simulink model "ControlEngineeringSimulink"  (R2020a)
settings: Solver=FixedStepAuto  StartTime=0.0  StopTime=50  FixedStep=1/8000  RelTol=1e-3
values from neighbouring files (symbols this model uses):
  A = [0 1 0 0 ... (first row only)    [ControllerToProject.m]
  B = [0 0 ... (first row only)    [ControllerToProject.m]
  C = [1 0 0 0 ... (first row only)    [ControllerToProject.m]
  g = 9.81    [ControllerToProject.m]    (also in Parameters.m = 9.82)
  l = 0.36022    [ControllerToProject.m]    (also in Parameters.m = 0.35)
  mc = 0.9+0.1    (= 1)    [ControllerToProject.m]    (also in Parameters.m = 0.9)
  mp = 0.08887    [ControllerToProject.m]    (also in Parameters.m = 0.1)
undefined symbols (not defined in the file or in its folder): bc, F, Fi, L, M, sigbuilder_block
libraries: simulink x4
settings Model: Creator=Emil  LastModifiedBy=Emil
settings SolverCC: ZeroCrossAlgorithm=Adaptive  AlgebraicLoopSolver=LineSearch
settings DebuggingCC: IgnoredZcDiagnostic=none

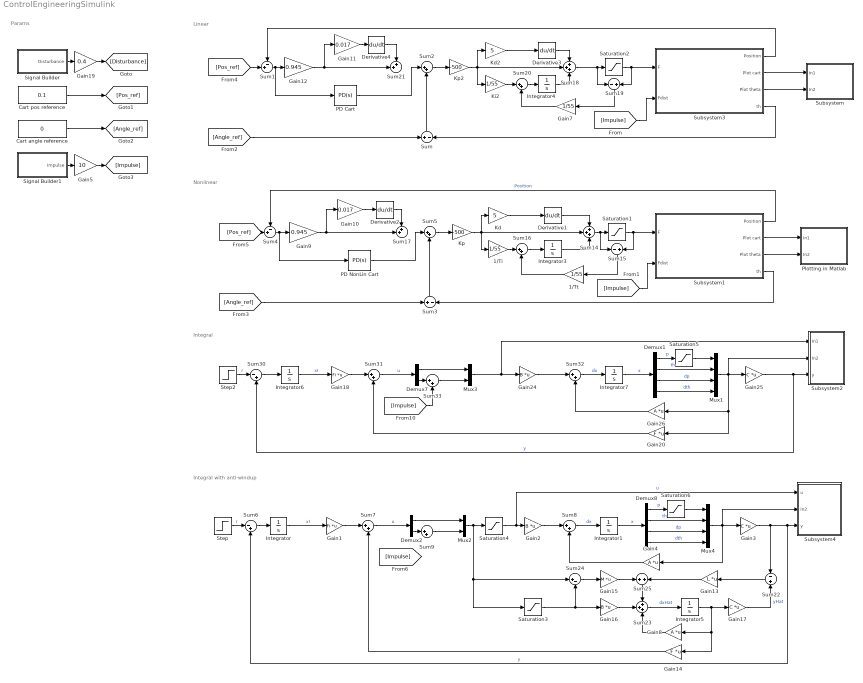
== system ControlEngineeringSimulink ==
  note: Params
  note: Nonlinear
  note: Linear
  note: Integral with anti-windup
  note: Integral
  1/Ti : Gain  Gain=1/55
  1/Tt : Gain  Gain=1/55
  Cart angle reference : Constant  Value=0
  Cart pos reference : Constant  Value=0.1
  Demux1 : Demux
  Demux2 : Demux  Outputs=2
  Demux7 : Demux  Outputs=2
  Demux8 : Demux
  Derivative{1..4} (4 alike) : Derivative
  Gain1 : Gain  Gain=Fi  Multiplication=Matrix(K*u)
  Gain10 : Gain  Gain=0.017
  Gain11 : Gain  Gain=0.017
  Gain12 : Gain  Gain=0.945
  Gain13 : Gain  Gain=L  Multiplication=Matrix(K*u)
  Gain14 : Gain  Gain=F  Multiplication=Matrix(K*u)
  Gain15 : Gain  Gain=M  Multiplication=Matrix(K*u)
  Gain16 : Gain  Gain=B  Multiplication=Matrix(K*u)
  Gain17 : Gain  Gain=C  Multiplication=Matrix(K*u)
  Gain18 : Gain  Gain=Fi  Multiplication=Matrix(K*u)
  Gain19 : Gain  Gain=0.4
  Gain2 : Gain  Gain=B  Multiplication=Matrix(K*u)
  Gain20 : Gain  Gain=F  Multiplication=Matrix(K*u)
  Gain24 : Gain  Gain=B  Multiplication=Matrix(K*u)
  Gain25 : Gain  Gain=C  Multiplication=Matrix(K*u)
  Gain26 : Gain  Gain=A  Multiplication=Matrix(K*u)
  Gain3 : Gain  Gain=C  Multiplication=Matrix(K*u)
  Gain4 : Gain  Gain=A  Multiplication=Matrix(K*u)
  Gain5 : Gain  Gain=10
  Gain7 : Gain  Gain=1/55
  Gain8 : Gain  Gain=A  Multiplication=Matrix(K*u)
  Gain9 : Gain  Gain=0.945
  Integrator{,1,3..7} (7 alike) : Integrator
  Kd : Gain  Gain=5
  Kd2 : Gain  Gain=5
  Ki2 : Gain  Gain=1/55
  Kp : Gain  Gain=-500
  Kp2 : Gain  Gain=-500
  Mux1 : Mux
  Mux2 : Mux  Inputs=2
  Mux3 : Mux  Inputs=2
  Mux4 : Mux
  PD Cart : simulink/Continuous/PID Controller  Controller=PD  Form=Ideal  TimeDomain=Continuous-time  UseExternalTs=off  SampleTime=-1  IntegratorMethod=Forward Euler  FilterMethod=Forward Euler  ControllerParametersSource=internal  P=0.945  I=0  D=0.017  UseFilter=on  N=20  TunerSelectOption=Transfer Function Based (PID Tuner App)  InitialConditionSource=internal  InitialConditionForIntegrator=0  InitialConditionForFilter=0  DifferentiatorICPrevScaledInput=0  ExternalReset=none  TrackingMode=off  Kt=1  LimitOutput=off  UpperSaturationLimit=inf  LowerSaturationLimit=-inf  LinearizeAsGain=on  AntiWindupMode=none  Kb=1  POutMin=[]  POutMax=[]  IOutMin=[]  IOutMax=[]  DOutMin=[]  DOutMax=[]  NOutMin=[]  NOutMax=[]  SumOutMin=[]  SumOutMax=[]  SaturationOutMin=[]  SaturationOutMax=[]  PParamMin=[]  PParamMax=[]  IParamMin=[]  IParamMax=[]  DParamMin=[]  DParamMax=[]  NParamMin=[]  NParamMax=[]  KbParamMin=[]  KbParamMax=[]  KtParamMin=[]  KtParamMax=[]  KbOutMin=[]  KbOutMax=[]  KtOutMin=[]  KtOutMax=[]  IntegratorOutMin=[]  IntegratorOutMax=[]  FilterOutMin=[]  FilterOutMax=[]  SumI1OutMin=[]  SumI1OutMax=[]  SumI2OutMin=[]  SumI2OutMax=[]  SumI3OutMin=[]  SumI3OutMax=[]  SumI4OutMin=[]  SumI4OutMax=[]  SumDOutMin=[]  SumDOutMax=[]  DifferentiatorOutMin=[]  DifferentiatorOutMax=[]  FilterDiffOutCoefMin=[]  FilterDiffOutCoefMax=[]  ReciprocalOutMin=[]  ReciprocalOutMax=[]  SumDenOutMin=[]  SumDenOutMax=[]  SumNumOutMin=[]  SumNumOutMax=[]  DivideOutMin=[]  DivideOutMax=[]  UdiffTsProdOutMin=[]  UdiffTsProdOutMax=[]  NTsProdOutMin=[]  NTsProdOutMax=[]  UintegralTsProdOutMin=[]  UintegralTsProdOutMax=[]  UngainTsProdOutMin=[]  UngainTsProdOutMax=[]  IntegratorContinuousStateAttributes=''  IntegratorStateMustResolveToSignalObject=off  IntegratorRTWStateStorageClass=Auto  FilterContinuousStateAttributes=''  FilterStateMustResolveToSignalObject=off  FilterRTWStateStorageClass=Auto  ParallelPVariant=Passthrough  IdealPVariant=InternalParameters  IVariant=Disabled  DVariant=InternalParameters  IntegratorVariant=Disabled  SatVariant=Disabled  AWVariant=Disabled  PCopyVariant=Disabled  TRVariant=Disabled  FdbkBlocksVariant=Forward  IdealPFdbkVariant=Disabled  SatFdbkVariant=Disabled  DerivativeFilterVariant=ContFilter  NVariant=InternalParameters  NCopyVariant=Disabled  FilterICVariant=InternalICsFilter  IntegratorICVariant=Disabled  ExternalResetVariant=Disabled  TRSumVariant=Passthrough  SumFdbkVariant=Disabled  SumVariant=Sum_PD  TsampFilterVariant=InternalTs  TsampNgainVariant=Passthrough  TsampIntegralVariant=Disabled_SignalSpec
  PD NonLin Cart : simulink/Continuous/PID Controller  Controller=PD  Form=Ideal  TimeDomain=Continuous-time  UseExternalTs=off  SampleTime=-1  IntegratorMethod=Forward Euler  FilterMethod=Forward Euler  ControllerParametersSource=internal  P=0.945  I=0  D=0.017  UseFilter=on  N=20  TunerSelectOption=Transfer Function Based (PID Tuner App)  InitialConditionSource=internal  InitialConditionForIntegrator=0  InitialConditionForFilter=0  DifferentiatorICPrevScaledInput=0  ExternalReset=none  TrackingMode=off  Kt=1  LimitOutput=off  UpperSaturationLimit=inf  LowerSaturationLimit=-inf  LinearizeAsGain=on  AntiWindupMode=none  Kb=1  POutMin=[]  POutMax=[]  IOutMin=[]  IOutMax=[]  DOutMin=[]  DOutMax=[]  NOutMin=[]  NOutMax=[]  SumOutMin=[]  SumOutMax=[]  SaturationOutMin=[]  SaturationOutMax=[]  PParamMin=[]  PParamMax=[]  IParamMin=[]  IParamMax=[]  DParamMin=[]  DParamMax=[]  NParamMin=[]  NParamMax=[]  KbParamMin=[]  KbParamMax=[]  KtParamMin=[]  KtParamMax=[]  KbOutMin=[]  KbOutMax=[]  KtOutMin=[]  KtOutMax=[]  IntegratorOutMin=[]  IntegratorOutMax=[]  FilterOutMin=[]  FilterOutMax=[]  SumI1OutMin=[]  SumI1OutMax=[]  SumI2OutMin=[]  SumI2OutMax=[]  SumI3OutMin=[]  SumI3OutMax=[]  SumI4OutMin=[]  SumI4OutMax=[]  SumDOutMin=[]  SumDOutMax=[]  DifferentiatorOutMin=[]  DifferentiatorOutMax=[]  FilterDiffOutCoefMin=[]  FilterDiffOutCoefMax=[]  ReciprocalOutMin=[]  ReciprocalOutMax=[]  SumDenOutMin=[]  SumDenOutMax=[]  SumNumOutMin=[]  SumNumOutMax=[]  DivideOutMin=[]  DivideOutMax=[]  UdiffTsProdOutMin=[]  UdiffTsProdOutMax=[]  NTsProdOutMin=[]  NTsProdOutMax=[]  UintegralTsProdOutMin=[]  UintegralTsProdOutMax=[]  UngainTsProdOutMin=[]  UngainTsProdOutMax=[]  IntegratorContinuousStateAttributes=''  IntegratorStateMustResolveToSignalObject=off  IntegratorRTWStateStorageClass=Auto  FilterContinuousStateAttributes=''  FilterStateMustResolveToSignalObject=off  FilterRTWStateStorageClass=Auto  ParallelPVariant=Passthrough  IdealPVariant=InternalParameters  IVariant=Disabled  DVariant=InternalParameters  IntegratorVariant=Disabled  SatVariant=Disabled  AWVariant=Disabled  PCopyVariant=Disabled  TRVariant=Disabled  FdbkBlocksVariant=Forward  IdealPFdbkVariant=Disabled  SatFdbkVariant=Disabled  DerivativeFilterVariant=ContFilter  NVariant=InternalParameters  NCopyVariant=Disabled  FilterICVariant=InternalICsFilter  IntegratorICVariant=Disabled  ExternalResetVariant=Disabled  TRSumVariant=Passthrough  SumFdbkVariant=Disabled  SumVariant=Sum_PD  TsampFilterVariant=InternalTs  TsampNgainVariant=Passthrough  TsampIntegralVariant=Disabled_SignalSpec
  Plotting in Matlab : Subsystem
  Saturation{1..4} (4 alike) : Saturate  UpperLimit=50  LowerLimit=-50
  Saturation5 : Saturate  UpperLimit=0.8  LowerLimit=-0.8
  Saturation6 : Saturate  UpperLimit=0.8  LowerLimit=-0.8
  Signal Builder : Subsystem  Tag=STV Subsys  LoadFcn=sigbuilder_block('load');  StartFcn=sigbuilder_block('start');  StopFcn=sigbuilder_block('stop');  ClipboardFcn=sigbuilder_block('clipboard');  mask(Sigbuilder block){tuvar=[0:10]}
      mask help: Simulink:masks:SigbuilderBlock_MD
      mask init:
      | if ~strcmp(get_param(bdroot(gcbh),'SimulationStatus'),'stopped') tuvar = sigbuilder_block('maskInit'); end
      settings: CopyFcn=sigbuilder_block('copy');  DeleteFcn=sigbuilder_block('delete');  ModelCloseFcn=sigbuilder_block('modelClose');  PreSaveFcn=sigbuilder_block('preSave');  PauseFcn=sigbuilder_block('pause');  ContinueFcn=sigbuilder_block('continue');  NameChangeFcn=sigbuilder_block('namechange');  OpenFcn=sigbuilder_block('open',[3.75 670.5 818.25 342 ]);  CloseFcn=sigbuilder_block('close');
      mask Display: plot(0, 0, 100, 100,[2, 2, 32, 32, 2], [68, 8, 8, 68, 68],[32, 2], [38, 38], [32, 19, 2],[53, 60, 44], [32, 17, 17, 2],[16, 16, 31, 31]);txt = getActiveGroup(gcbh);text(2, 100, txt,'verticalAlignment', 'top');
  Signal Builder1 : Subsystem  Tag=STV Subsys  LoadFcn=sigbuilder_block('load');  StartFcn=sigbuilder_block('start');  StopFcn=sigbuilder_block('stop');  ClipboardFcn=sigbuilder_block('clipboard');  mask(Sigbuilder block){tuvar=[0:10]}
      mask help: Simulink:masks:SigbuilderBlock_MD
      mask init:
      | if ~strcmp(get_param(bdroot(gcbh),'SimulationStatus'),'stopped') tuvar = sigbuilder_block('maskInit'); end
      settings: CopyFcn=sigbuilder_block('copy');  DeleteFcn=sigbuilder_block('delete');  ModelCloseFcn=sigbuilder_block('modelClose');  PreSaveFcn=sigbuilder_block('preSave');  PauseFcn=sigbuilder_block('pause');  ContinueFcn=sigbuilder_block('continue');  NameChangeFcn=sigbuilder_block('namechange');  OpenFcn=sigbuilder_block('open',[437.6 199.2 550.4 400 ]);  CloseFcn=sigbuilder_block('close');
      mask Display: plot(0, 0, 100, 100,[2, 2, 32, 32, 2], [68, 8, 8, 68, 68],[32, 2], [38, 38], [32, 19, 2],[53, 60, 44], [32, 17, 17, 2],[16, 16, 31, 31]);txt = getActiveGroup(gcbh);text(2, 100, txt,'verticalAlignment', 'top');
  Step : Step  Time=0  Before=[0, 0]  After=[0, 0.1]  SampleTime=0
  Step2 : Step  Time=0  Before=[0, 0]  After=[0, 0.1]  SampleTime=0
  Subsystem : Subsystem
  Subsystem1 : Subsystem
      mask Display: image('System.png'); % Use "Edit Image" on toolstrip to change.
  Subsystem2 : Subsystem
  Subsystem3 : Subsystem
      mask Display: image('System.png'); % Use "Edit Image" on toolstrip to change.
  Subsystem4 : Subsystem
  Sum : Sum  Inputs=+-
  Sum1 : Sum  Inputs=-+|
  Sum14 : Sum  Inputs=+++
  Sum15 : Sum  Inputs=-+
  Sum{2,5,7..9,16,20,31..33} (10 alike) : Sum  Inputs=|++
  Sum17 : Sum  Inputs=++|
  Sum18 : Sum  Inputs=+++
  Sum19 : Sum  Inputs=-+
  Sum21 : Sum  Inputs=++|
  Sum22 : Sum  Inputs=-+
  Sum23 : Sum  Inputs=+++
  Sum24 : Sum  Inputs=|+-
  Sum25 : Sum
  Sum3 : Sum  Inputs=+-
  Sum30 : Sum  Inputs=|-+
  Sum4 : Sum  Inputs=-+|
  Sum6 : Sum  Inputs=|-+
  wires:
  Subsystem3/1(Position) -> Sum1/1
  Subsystem3/4(th) -> Sum/2
  [Angle_ref] -> Sum/1
  [Pos_ref] -> Sum1/2
  Sum/1 -> Sum2/2
  [Pos_ref] -> Sum4/2
  [Angle_ref] -> Sum3/1
  Sum3/1 -> Sum5/2
  Subsystem1/1(Position) -> Sum4/1  "Position"
  Subsystem1/4(th) -> Sum3/2
  Cart pos reference/1 -> [Pos_ref]
  Cart angle reference/1 -> [Angle_ref]
  Sum6/1 -> Integrator/1
  Gain3/1 -> Sum22/1, Sum6/2, Subsystem4/3(y)  "y"
  Gain1/1 -> Sum7/1
  Gain2/1 -> Sum8/1
  Step/1 -> Sum6/1  "r"
  Gain4/1 -> Sum8/2
  Mux4/1 -> Gain4/1, Subsystem4/2(In2), Gain3/1
  Integrator/1 -> Gain1/1  "xI"
  Sum9/1 -> Mux2/2
  Sum7/1 -> Demux2/1  "u"
  Mux2/1 -> Saturation3/1, Sum24/1, Saturation4/1
  Demux2/1 -> Mux2/1
  Sum8/1 -> Integrator1/1  "dx"
  Kp/1 -> 1/Ti/1, Sum14/2, Kd/1
  Integrator3/1 -> Sum14/3
  Derivative1/1 -> Sum14/1
  Saturation1/1 -> Subsystem1/1(F), Sum15/2
  Kd/1 -> Derivative1/1
  1/Ti/1 -> Sum16/1
  Sum16/1 -> Integrator3/1
  Derivative2/1 -> Sum17/1
  Sum14/1 -> Sum15/1, Saturation1/1
  Sum15/1 -> 1/Tt/1
  1/Tt/1 -> Sum16/2
  Gain9/1 -> Gain10/1, Sum17/2
  Sum19/1 -> Gain7/1
  Gain7/1 -> Sum20/2
  Sum18/1 -> Sum19/1, Saturation2/1
  Sum2/1 -> Kp2/1
  Kd2/1 -> Derivative3/1
  Ki2/1 -> Sum20/1
  Sum20/1 -> Integrator4/1
  Saturation2/1 -> Sum19/2, Subsystem3/1(F)
  Integrator4/1 -> Sum18/3
  Derivative3/1 -> Sum18/1
  Kp2/1 -> Ki2/1, Sum18/2, Kd2/1
  Gain11/1 -> Derivative4/1
  Gain12/1 -> Sum21/2, Gain11/1
  Derivative4/1 -> Sum21/1
  Gain15/1 -> Sum25/1
  Integrator5/1 -> Gain14/1, Gain8/1, Gain17/1
  Saturation3/1 -> Gain16/1, Sum24/2
  Gain14/1 -> Sum7/2
  Saturation4/1 -> Subsystem4/1(u), Gain2/1  "u"
  Sum24/1 -> Gain15/1
  Gain13/1 -> Sum25/2
  Gain17/1 -> Sum22/2  "yHat"
  Sum25/1 -> Sum23/1
  Sum23/1 -> Integrator5/1  "dxHat"
  Gain8/1 -> Sum23/3
  Gain16/1 -> Sum23/2
  Sum22/1 -> Gain13/1
  Gain10/1 -> Derivative2/1
  Sum5/1 -> Kp/1
  Sum4/1 -> PD NonLin Cart/1, Gain9/1
  Demux1/1 -> Saturation5/1  "p"
  Demux1/3 -> Mux1/3  "dp"
  Integrator7/1 -> Demux1/1  "x"
  Gain25/1 -> Sum30/2, Subsystem2/3(y)  "y"
  Gain26/1 -> Sum32/2
  Demux7/2 -> Sum33/1
  Gain24/1 -> Sum32/1
  Sum33/1 -> Mux3/2
  Sum31/1 -> Demux7/1  "u"
  Sum30/1 -> Integrator6/1
  Demux1/4 -> Mux1/4  "dth"
  Mux3/1 -> Subsystem2/1(In1), Gain24/1
  Mux1/1 -> Gain20/1, Gain26/1, Subsystem2/2(In2), Gain25/1
  Integrator6/1 -> Gain18/1  "xI"
  Sum32/1 -> Integrator7/1  "dx"
  Demux7/1 -> Mux3/1
  Gain18/1 -> Sum31/1
  Step2/1 -> Sum30/1  "r"
  Gain20/1 -> Sum31/2
  Saturation5/1 -> Mux1/1
  Demux1/2 -> Mux1/2  "th"
  Demux8/4 -> Mux4/4  "dth"
  Demux8/3 -> Mux4/3  "dp"
  Demux8/2 -> Mux4/2  "th"
  Integrator1/1 -> Demux8/1  "x"
  Saturation6/1 -> Mux4/1
  Demux8/1 -> Saturation6/1  "p"
  Signal Builder/1(Disturbance) -> Gain19/1
  Gain19/1 -> [Disturbance]
  Demux2/2 -> Sum9/1
  Signal Builder1/1(Impulse) -> Gain5/1
  Gain5/1 -> [Impulse]
  [Impulse] -> Subsystem3/2(Fdist)
  [Impulse] -> Subsystem1/2(Fdist)
  Subsystem1/2(Plot cart) -> Plotting in Matlab/1(In1)
  Subsystem1/3(Plot theta) -> Plotting in Matlab/2(In2)
  Subsystem3/2(Plot cart) -> Subsystem/1(In1)
  Subsystem3/3(Plot theta) -> Subsystem/2(In2)
  Sum1/1 -> PD Cart/1, Gain12/1
  PD Cart/1 -> Sum2/1
  PD NonLin Cart/1 -> Sum5/1
  [Impulse] -> Sum33/2

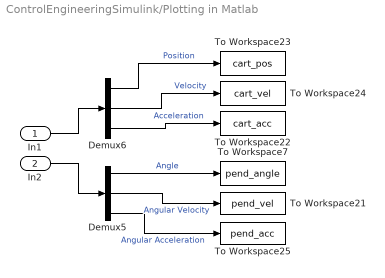
== system ControlEngineeringSimulink/Plotting in Matlab ==
  In1 : Inport
  In2 : Inport  Port=2
  Demux5 : Demux  Outputs=3
  Demux6 : Demux  Outputs=3
  To Workspace21 : ToWorkspace  VariableName=pend_vel  SaveFormat=Timeseries  SampleTime=-1
  To Workspace22 : ToWorkspace  VariableName=cart_acc  SaveFormat=Timeseries  SampleTime=-1
  To Workspace23 : ToWorkspace  VariableName=cart_pos  SaveFormat=Timeseries  SampleTime=-1
  To Workspace24 : ToWorkspace  VariableName=cart_vel  SaveFormat=Timeseries  SampleTime=-1
  To Workspace25 : ToWorkspace  VariableName=pend_acc  SaveFormat=Timeseries  SampleTime=-1
  To Workspace7 : ToWorkspace  VariableName=pend_angle  SaveFormat=Timeseries  SampleTime=-1
  wires:
  In1/1 -> Demux6/1
  Demux5/1 -> To Workspace7/1  "Angle"
  In2/1 -> Demux5/1
  Demux5/2 -> To Workspace21/1  "Angular Velocity"
  Demux6/1 -> To Workspace23/1  "Position"
  Demux5/3 -> To Workspace25/1  "Angular Acceleration"
  Demux6/2 -> To Workspace24/1  "Velocity"
  Demux6/3 -> To Workspace22/1  "Acceleration"

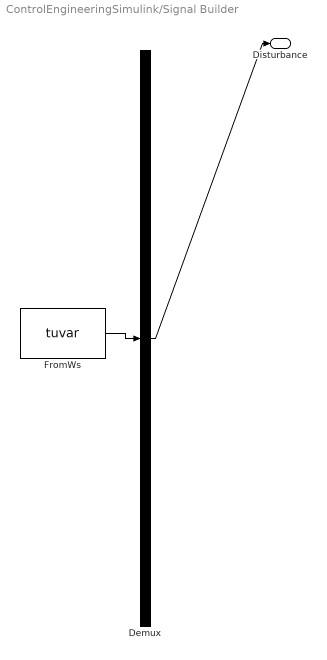
== system ControlEngineeringSimulink/Signal Builder ==
  Demux : Demux  Tag=STV Demux  Outputs=1
      settings: DisplayOption=none
  FromWs : FromWorkspace  Tag=STV FromWs  VariableName=tuvar
      SigBuilderData=|
      | common.afterFinalStr = 'Extrapolate'
      | common.sampleTime = 0
      | dataSet.timeRange = [0 10]
      | dataSet.name = 'Group 1'
      | sbobj.Groups.Name = 'Group 1'
      | sbobj.Groups.Signals.Name = 'Disturbance'
      | sbobj.Groups.Signals.XData = [0 0.25 0.5 0.75 1 1.25 1.5 1.75 2 2.25 2.5 2.75 3 3.25 3.5 3.75 4 4.25 4.5 4.75 5 5.25 5.5 5.75 6 6.25 6.5 6.75 7 7.25 7.5 7.75 8 8.25 8.5 8.75 9 9.25 9.5 9.75 10]
      | sbobj.Groups.Signals.YData = [0 0 0 0 0 0 0 0 0 0 0 -2.77555756156e-17 -0.002 0.063 0.002 -0.03 -0.05 -0.05 0.01 -0.146 0.16 0.08 0.1 0.089 0.193 0.06 0.02 -2.7756e-18 -0.022 -0.034 -0.099 -0.084 -0.01 -0.02 -0.051 -0.045 0.02 0.02 0.176 -2.7756e-18 -2.77555756156e-17]
  Disturbance : Outport  Tag=STV Outport
  wires:
  FromWs/1 -> Demux/1
  Demux/1 -> Disturbance/1

== system ControlEngineeringSimulink/Signal Builder1 ==
  Demux : Demux  Tag=STV Demux  Outputs=1
      settings: DisplayOption=none
  FromWs : FromWorkspace  Tag=STV FromWs  VariableName=tuvar
      SigBuilderData=|
      | common.afterFinalStr = 'Extrapolate'
      | common.sampleTime = 0
      | dataSet.timeRange = [0 10]
      | dataSet.name = 'Group 1'
      | sbobj.Groups.Name = 'Group 1'
      | sbobj.Groups.Signals.Name = 'Impulse'
      | sbobj.Groups.Signals.XData = [0 0.1 0.2 10]
      | sbobj.Groups.Signals.YData = [0 0.01 0 0]
  Impulse : Outport  Tag=STV Outport
  wires:
  FromWs/1 -> Demux/1
  Demux/1 -> Impulse/1

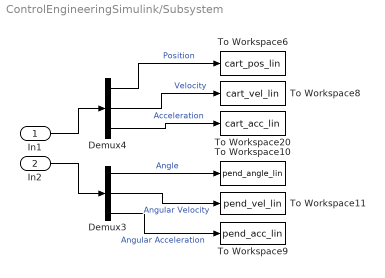
== system ControlEngineeringSimulink/Subsystem ==
  In1 : Inport
  In2 : Inport  Port=2
  Demux3 : Demux  Outputs=3
  Demux4 : Demux  Outputs=3
  To Workspace10 : ToWorkspace  VariableName=pend_angle_lin  SaveFormat=Timeseries  SampleTime=-1
  To Workspace11 : ToWorkspace  VariableName=pend_vel_lin  SaveFormat=Timeseries  SampleTime=-1
  To Workspace20 : ToWorkspace  VariableName=cart_acc_lin  SaveFormat=Timeseries  SampleTime=-1
  To Workspace6 : ToWorkspace  VariableName=cart_pos_lin  SaveFormat=Timeseries  SampleTime=-1
  To Workspace8 : ToWorkspace  VariableName=cart_vel_lin  SaveFormat=Timeseries  SampleTime=-1
  To Workspace9 : ToWorkspace  VariableName=pend_acc_lin  SaveFormat=Timeseries  SampleTime=-1
  wires:
  Demux4/2 -> To Workspace8/1  "Velocity"
  Demux4/1 -> To Workspace6/1  "Position"
  In1/1 -> Demux4/1
  In2/1 -> Demux3/1
  Demux3/2 -> To Workspace11/1  "Angular Velocity"
  Demux3/1 -> To Workspace10/1  "Angle"
  Demux3/3 -> To Workspace9/1  "Angular Acceleration"
  Demux4/3 -> To Workspace20/1  "Acceleration"

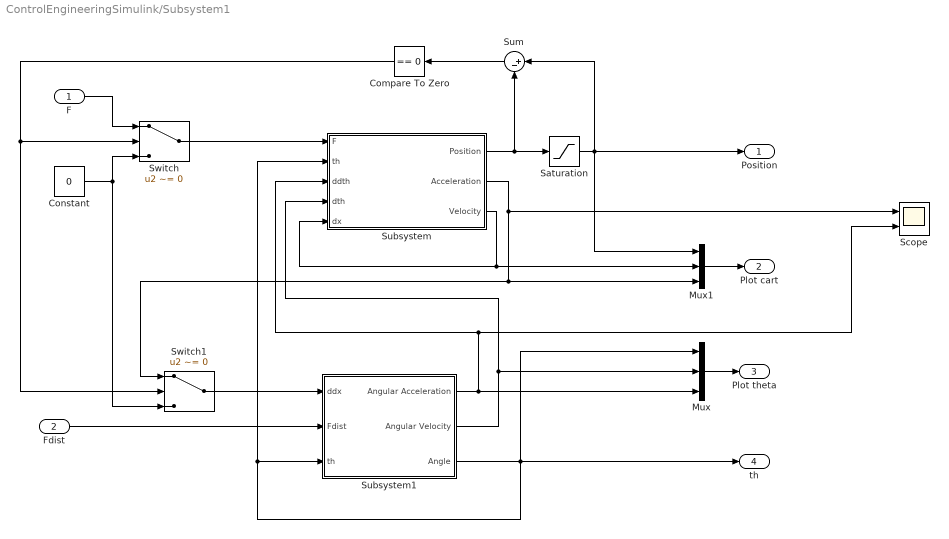
== system ControlEngineeringSimulink/Subsystem1 ==
  F : Inport
  Fdist : Inport  Port=2
  Compare To Zero : simulink/Logic and Bit Operations/Compare To Zero  relop===  OutDataTypeStr=boolean
  Constant : Constant  Value=0
  Mux : Mux  Inputs=3
  Mux1 : Mux  Inputs=3
  Saturation : Saturate  UpperLimit=0.8  LowerLimit=-0.8
  Scope : Scope  NumInputPorts=2
  Subsystem : Subsystem
      mask Display: image('Cart.png'); % Use "Edit Image" on toolstrip to change.
  Subsystem1 : Subsystem
      mask Display: image('Pendulum.png'); % Use "Edit Image" on toolstrip to change.
  Sum : Sum  Inputs=|+-
  Switch : Switch  Criteria=u2 ~= 0
  Switch1 : Switch  Criteria=u2 ~= 0
  Position : Outport
  Plot cart : Outport  Port=2
  Plot theta : Outport  Port=3
  th : Outport  Port=4
  wires:
  Fdist/1 -> Subsystem1/2(Fdist)
  Subsystem/3(Velocity) -> Mux1/2, Subsystem/5(dx)
  Sum/1 -> Compare To Zero/1
  Subsystem/1(Position) -> Saturation/1, Sum/2
  F/1 -> Switch/1
  Constant/1 -> Switch1/3, Switch/3
  Compare To Zero/1 -> Switch1/2, Switch/2
  Switch/1 -> Subsystem/1(F)
  Switch1/1 -> Subsystem1/1(ddx)
  Mux/1 -> Plot theta/1
  Mux1/1 -> Plot cart/1
  Subsystem1/3(Angle) -> Mux/1, th/1, Subsystem/2(th), Subsystem1/3(th)
  Saturation/1 -> Mux1/1, Sum/1, Position/1
  Subsystem/2(Acceleration) -> Switch1/1, Mux1/3, Scope/1
  Subsystem1/1(Angular Acceleration) -> Mux/3, Scope/2, Subsystem/3(ddth)
  Subsystem1/2(Angular Velocity) -> Mux/2, Subsystem/4(dth)

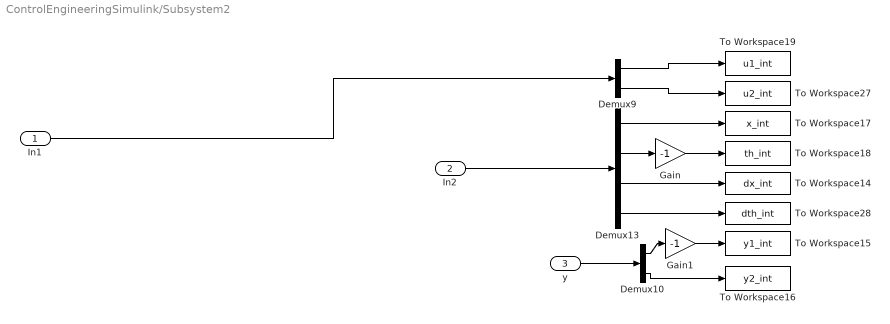
== system ControlEngineeringSimulink/Subsystem2 ==
  In1 : Inport
  In2 : Inport  Port=2
  y : Inport  Port=3
  Demux10 : Demux  Outputs=2
  Demux13 : Demux
  Demux9 : Demux  Outputs=2
  Gain : Gain  Gain=-1
  Gain1 : Gain  Gain=-1
  To Workspace14 : ToWorkspace  VariableName=dx_int  SaveFormat=Timeseries  SampleTime=-1
  To Workspace15 : ToWorkspace  VariableName=y1_int  SaveFormat=Timeseries  SampleTime=-1
  To Workspace16 : ToWorkspace  VariableName=y2_int  SaveFormat=Timeseries  SampleTime=-1
  To Workspace17 : ToWorkspace  VariableName=x_int  SaveFormat=Timeseries  SampleTime=-1
  To Workspace18 : ToWorkspace  VariableName=th_int  SaveFormat=Timeseries  SampleTime=-1
  To Workspace19 : ToWorkspace  VariableName=u1_int  SaveFormat=Timeseries  SampleTime=-1
  To Workspace27 : ToWorkspace  VariableName=u2_int  SaveFormat=Timeseries  SampleTime=-1
  To Workspace28 : ToWorkspace  VariableName=dth_int  SaveFormat=Timeseries  SampleTime=-1
  wires:
  Demux13/1 -> To Workspace17/1
  In1/1 -> Demux9/1
  Demux13/2 -> Gain/1
  Demux13/3 -> To Workspace14/1
  Demux10/1 -> Gain1/1
  Demux9/1 -> To Workspace19/1
  Demux9/2 -> To Workspace27/1
  Demux13/4 -> To Workspace28/1
  y/1 -> Demux10/1
  In2/1 -> Demux13/1
  Gain/1 -> To Workspace18/1
  Demux10/2 -> To Workspace16/1
  Gain1/1 -> To Workspace15/1

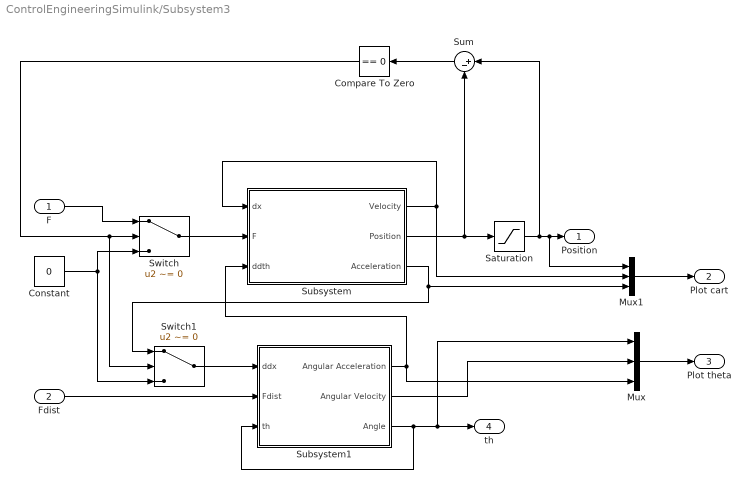
== system ControlEngineeringSimulink/Subsystem3 ==
  F : Inport
  Fdist : Inport  Port=2
  Compare To Zero : simulink/Logic and Bit Operations/Compare To Zero  relop===  OutDataTypeStr=boolean
  Constant : Constant  Value=0
  Mux : Mux  Inputs=3
  Mux1 : Mux  Inputs=3
  Saturation : Saturate  UpperLimit=0.8  LowerLimit=-0.8
  Subsystem : Subsystem
      mask Display: image('Cart.png'); % Use "Edit Image" on toolstrip to change.
  Subsystem1 : Subsystem
      mask Display: image('Pendulum.png'); % Use "Edit Image" on toolstrip to change.
  Sum : Sum  Inputs=|+-
  Switch : Switch  Criteria=u2 ~= 0
  Switch1 : Switch  Criteria=u2 ~= 0
  Position : Outport
  Plot cart : Outport  Port=2
  Plot theta : Outport  Port=3
  th : Outport  Port=4
  wires:
  F/1 -> Switch/1
  Fdist/1 -> Subsystem1/2(Fdist)
  Subsystem/2(Position) -> Saturation/1, Sum/2
  Sum/1 -> Compare To Zero/1
  Constant/1 -> Switch1/3, Switch/3
  Compare To Zero/1 -> Switch1/2, Switch/2
  Switch/1 -> Subsystem/2(F)
  Switch1/1 -> Subsystem1/1(ddx)
  Subsystem1/1(Angular Acceleration) -> Subsystem/3(ddth), Mux/3
  Mux1/1 -> Plot cart/1
  Subsystem/3(Acceleration) -> Switch1/1, Mux1/3
  Subsystem/1(Velocity) -> Mux1/2, Subsystem/1(dx)
  Saturation/1 -> Sum/1, Mux1/1, Position/1
  Mux/1 -> Plot theta/1
  Subsystem1/3(Angle) -> Mux/1, th/1, Subsystem1/3(th)
  Subsystem1/2(Angular Velocity) -> Mux/2

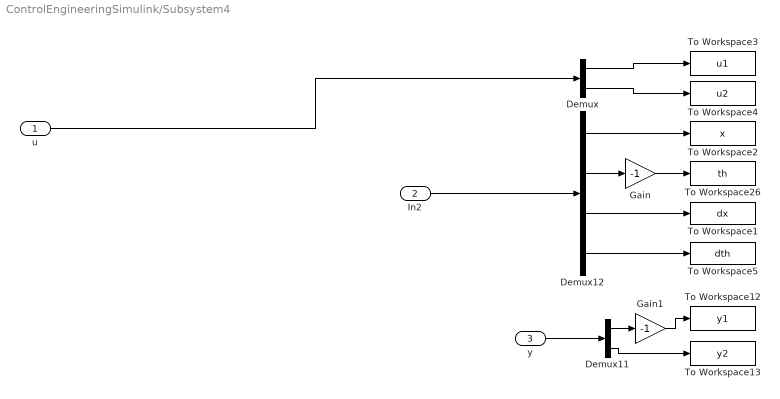
== system ControlEngineeringSimulink/Subsystem4 ==
  u : Inport
  In2 : Inport  Port=2
  y : Inport  Port=3
  Demux : Demux  Outputs=2
  Demux11 : Demux  Outputs=2
  Demux12 : Demux
  Gain : Gain  Gain=-1
  Gain1 : Gain  Gain=-1
  To Workspace1 : ToWorkspace  VariableName=dx  SaveFormat=Timeseries  SampleTime=-1
  To Workspace12 : ToWorkspace  VariableName=y1  SaveFormat=Timeseries  SampleTime=-1
  To Workspace13 : ToWorkspace  VariableName=y2  SaveFormat=Timeseries  SampleTime=-1
  To Workspace2 : ToWorkspace  VariableName=x  SaveFormat=Timeseries  SampleTime=-1
  To Workspace26 : ToWorkspace  VariableName=th  SaveFormat=Timeseries  SampleTime=-1
  To Workspace3 : ToWorkspace  VariableName=u1  SaveFormat=Timeseries  SampleTime=-1
  To Workspace4 : ToWorkspace  VariableName=u2  SaveFormat=Timeseries  SampleTime=-1
  To Workspace5 : ToWorkspace  VariableName=dth  SaveFormat=Timeseries  SampleTime=-1
  wires:
  y/1 -> Demux11/1
  u/1 -> Demux/1
  Demux11/1 -> Gain1/1
  Demux12/4 -> To Workspace5/1
  Demux/1 -> To Workspace3/1
  Demux12/1 -> To Workspace2/1
  Demux12/3 -> To Workspace1/1
  Demux12/2 -> Gain/1
  Demux/2 -> To Workspace4/1
  In2/1 -> Demux12/1
  Gain/1 -> To Workspace26/1
  Demux11/2 -> To Workspace13/1
  Gain1/1 -> To Workspace12/1

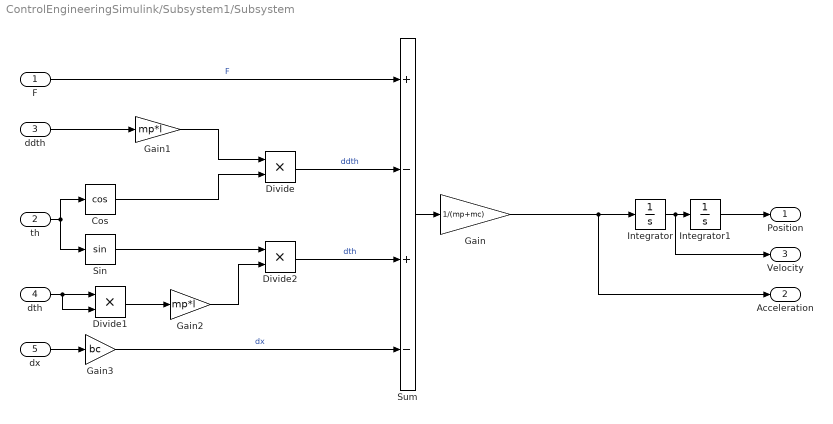
== system ControlEngineeringSimulink/Subsystem1/Subsystem ==
  F : Inport
  th : Inport  Port=2
  ddth : Inport  Port=3
  dth : Inport  Port=4
  dx : Inport  Port=5
  Cos : Trigonometry  Operator=cos
  Divide : Product  Inputs=**
  Divide1 : Product  Inputs=**
  Divide2 : Product  Inputs=**
  Gain : Gain  Gain=1/(mp+mc)
  Gain1 : Gain  Gain=mp*l
  Gain2 : Gain  Gain=mp*l
  Gain3 : Gain  Gain=bc
  Integrator : Integrator
  Integrator1 : Integrator
  Sin : Trigonometry
  Sum : Sum  Inputs=+-+-
  Position : Outport
  Acceleration : Outport  Port=2
  Velocity : Outport  Port=3
  wires:
  Sum/1 -> Gain/1
  th/1 -> Sin/1, Cos/1
  Integrator/1 -> Velocity/1, Integrator1/1
  Integrator1/1 -> Position/1
  ddth/1 -> Gain1/1
  Gain1/1 -> Divide/1
  Cos/1 -> Divide/2
  dth/1 -> Divide1/2, Divide1/1
  Divide1/1 -> Gain2/1
  Gain2/1 -> Divide2/2
  Sin/1 -> Divide2/1
  F/1 -> Sum/1  "F"
  Divide/1 -> Sum/2  "ddth"
  Divide2/1 -> Sum/3  "dth"
  dx/1 -> Gain3/1
  Gain/1 -> Acceleration/1, Integrator/1
  Gain3/1 -> Sum/4  "dx"

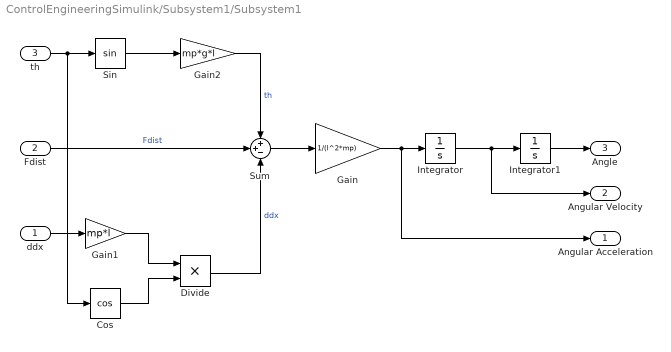
== system ControlEngineeringSimulink/Subsystem1/Subsystem1 ==
  ddx : Inport
  Fdist : Inport  Port=2
  th : Inport  Port=3
  Cos : Trigonometry  Operator=cos
  Divide : Product  Inputs=**
  Gain : Gain  Gain=1/(l^2*mp)
  Gain1 : Gain  Gain=mp*l
  Gain2 : Gain  Gain=mp*g*l
  Integrator : Integrator
  Integrator1 : Integrator
  Sin : Trigonometry
  Sum : Sum  Inputs=++-
  Angular Acceleration : Outport
  Angular Velocity : Outport  Port=2
  Angle : Outport  Port=3
  wires:
  Integrator/1 -> Angular Velocity/1, Integrator1/1
  Integrator1/1 -> Angle/1
  Gain/1 -> Angular Acceleration/1, Integrator/1
  Sum/1 -> Gain/1
  Fdist/1 -> Sum/2  "Fdist"
  ddx/1 -> Gain1/1
  th/1 -> Sin/1, Cos/1
  Gain1/1 -> Divide/1
  Cos/1 -> Divide/2
  Divide/1 -> Sum/3  "ddx"
  Sin/1 -> Gain2/1
  Gain2/1 -> Sum/1  "th"

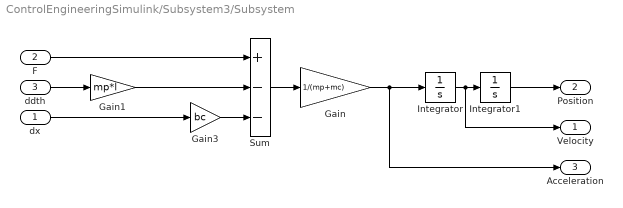
== system ControlEngineeringSimulink/Subsystem3/Subsystem ==
  dx : Inport
  F : Inport  Port=2
  ddth : Inport  Port=3
  Gain : Gain  Gain=1/(mp+mc)
  Gain1 : Gain  Gain=mp*l
  Gain3 : Gain  Gain=bc
  Integrator : Integrator
  Integrator1 : Integrator
  Sum : Sum  Inputs=+--
  Velocity : Outport
  Position : Outport  Port=2
  Acceleration : Outport  Port=3
  wires:
  Sum/1 -> Gain/1
  Gain/1 -> Integrator/1, Acceleration/1
  Integrator/1 -> Velocity/1, Integrator1/1
  Integrator1/1 -> Position/1
  ddth/1 -> Gain1/1
  F/1 -> Sum/1
  Gain1/1 -> Sum/2
  dx/1 -> Gain3/1
  Gain3/1 -> Sum/3

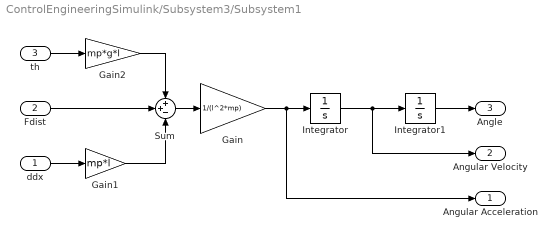
== system ControlEngineeringSimulink/Subsystem3/Subsystem1 ==
  ddx : Inport
  Fdist : Inport  Port=2
  th : Inport  Port=3
  Gain : Gain  Gain=1/(l^2*mp)
  Gain1 : Gain  Gain=mp*l
  Gain2 : Gain  Gain=mp*g*l
  Integrator : Integrator
  Integrator1 : Integrator
  Sum : Sum  Inputs=++-
  Angular Acceleration : Outport
  Angular Velocity : Outport  Port=2
  Angle : Outport  Port=3
  wires:
  Integrator/1 -> Angular Velocity/1, Integrator1/1
  Integrator1/1 -> Angle/1
  Gain/1 -> Angular Acceleration/1, Integrator/1
  Sum/1 -> Gain/1
  Fdist/1 -> Sum/2
  ddx/1 -> Gain1/1
  Gain1/1 -> Sum/3
  th/1 -> Gain2/1
  Gain2/1 -> Sum/1
